simulink model "hardware_atrias_raibert"  (R2014a)
settings: Solver=FixedStepDiscrete  StartTime=0.0  StopTime=inf  FixedStep=sample_time  RelTol=1e-3
InitFcn:
  | init_hardware_atrias_raibert;
undefined symbols (not defined in the file): A_lpf_accel, A_lpf_dtau, B1_lpf_accel, B1_lpf_dtau, B2_lpf_accel, B2_lpf_dtau, boom_mount_angle, boom_mount_to_center_diagonal, boom_mount_to_com, contact_threshold, control_start_time, desired_torso_angle, DiscIntNeverNeededParam, dt_thrust, dx_avg_desired, dx_avg_samples, F_thrust, fcut_contact, g, i_limit_lateral, j_segments, k_ff, k_placement, k_sea, kd_flight, kd_lateral, kd_leg_angle, kd_sea_torque_flight, kd_sea_torque_stance, kd_torso, kd_virtual, ki_lateral, kp_flight_max, kp_flight_min, kp_lateral, kp_leg_angle, kp_sea_torque_flight, kp_sea_torque_stance, kp_torso, kp_virtual, l0_virtual, l_boom, l_max, l_min, l_retract, l_seg, lambda1, lambda2, lateral_offset, lateral_torque_ramp_time, LEG_MTR_MAX_TORQUE, loaded_threshold, m_leg_motor, m_total, max_leg_angle, max_sagittal_loaded_torque, max_sagittal_unloaded_torque, max_torque_lateral, min_leg_angle, sagittal_torque_ramp_time ... (+7)
libraries: simulink x13
settings Model: xpc_rtwmakecfg_data=_xpcethercatlib_  BufferReuse=off  Creator=wmartin  LastModifiedBy=wmartin
settings SolverCC: EnableConcurrentExecution=on
settings DataIOCC: MaxDataPoints=1000000000  SaveFormat=StructureWithTime
settings OptimizationCC: BlockReduction=off  OptimizeBlockIOStorage=off  BufferReuse=off  GlobalBufferReuse=off  ExpressionFolding=off  ExpressionDepthLimit=2147483647  LocalBlockOutputs=off
settings DebuggingCC: UnderspecifiedInitializationDetection=Classic  StateNameClashWarn=warning
settings HardwareCC: ProdIntDivRoundTo=Zero  ProdEndianess=LittleEndian  ProdHWDeviceType=Generic->32-bit x86 compatible
settings RTWCC: SystemTargetFile=slrt.tlc  TemplateMakefile=slrt_default_tmf  Description=Simulink Real-Time  RTWVerbose=off  ProcessScript=slrt_make_rtw_hook  RTWCompilerOptimization=On
settings SimulinkRealTimeCC: GeneratePreprocessorConditionals=Disable all  EnableShiftOperators=on  RL32LogBufSizeModifier=100000000

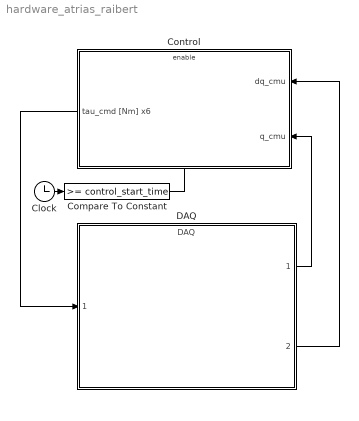
== system hardware_atrias_raibert ==
  Clock : Clock
  Compare To Constant : simulink/Logic and Bit Operations/Compare To Constant  relop=>=  const=control_start_time  OutDataTypeStr=boolean
  Control : Subsystem
  DAQ : ModelReference  ModelNameDialog=DAQ  SimulationMode=Normal  ModelReferenceVersion=1.1389  CopyOfModelName=DAQ  DefaultDataLogging=on
  wires:
  DAQ/1 -> Control/2(q_cmu)
  DAQ/2 -> Control/1(dq_cmu)
  Clock/1 -> Compare To Constant/1
  Compare To Constant/1 -> Control/Enable
  Control/1(tau_cmd [Nm] x6) -> DAQ/1

== system hardware_atrias_raibert/Control ==
  dq_cmu : Inport
  q_cmu : Inport  Port=2
  Enable : EnablePort  StatesWhenEnabling=reset
  Actuator Control : Subsystem
  Behavior Control : Subsystem
  tau_cmd [Nm] x6 : Outport  InitialOutput=[0 0 0 0 0 0]
  wires:
  Behavior Control/1(motor_torque_cmd) -> Actuator Control/1(tau_desired [Nm] x6)
  dq_cmu/1 -> Actuator Control/3(dq_cmu), Behavior Control/1(dq_cmu)
  Actuator Control/1(tau_cmd [Nm] x6) -> tau_cmd [Nm] x6/1
  q_cmu/1 -> Actuator Control/2(q_cmu), Behavior Control/2(q_cmu)

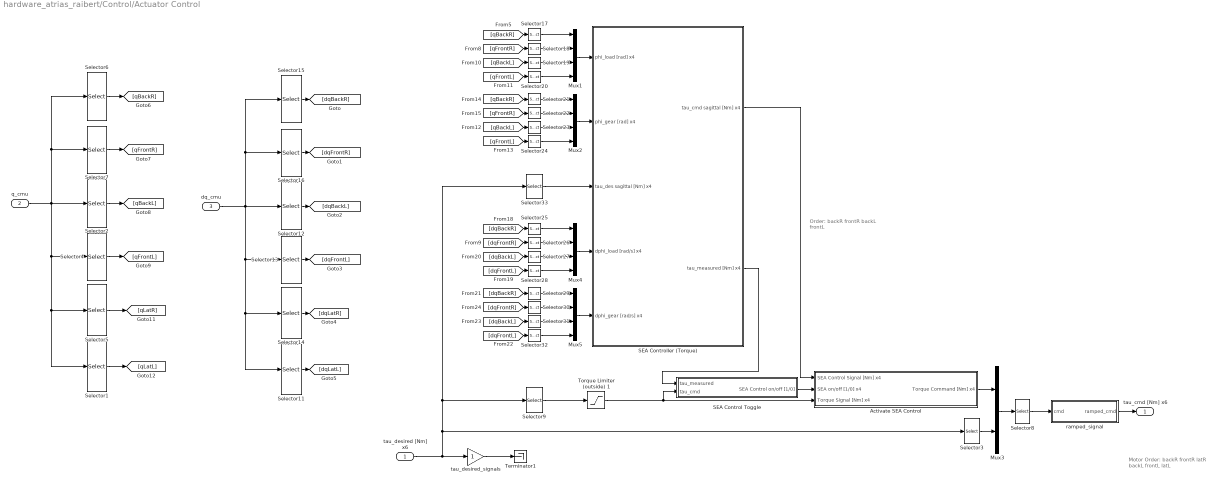
== system hardware_atrias_raibert/Control/Actuator Control ==
  note: Order:
      | backR
      | frontR
      | backL
      | frontL
  note: Motor Order:
      |
      | backR
      | frontR
      | latR
      | backL
      | frontL
      | latL
  tau_desired [Nm] x6 : Inport
  q_cmu : Inport  Port=2
  dq_cmu : Inport  Port=3
  Activate SEA Control : Subsystem
  Mux{1..2,4..5} (4 alike) : Mux
  Mux3 : Mux  Inputs=2
  SEA Control Toggle : Subsystem
  SEA Controller (Torque) : Subsystem
  Selector1 : Selector  InputPortWidth=13  Indices=[10]
  Selector11 : Selector  InputPortWidth=13  Indices=[10]
  Selector12 : Selector  InputPortWidth=13  Indices=[5 6]
  Selector13 : Selector  InputPortWidth=13  Indices=[7 8]
  Selector14 : Selector  InputPortWidth=13  Indices=[9]
  Selector15 : Selector  InputPortWidth=13  Indices=[1 2]
  Selector16 : Selector  InputPortWidth=13  Indices=[3 4]
  Selector{17..20,25..28} (8 alike) : Selector  InputPortWidth=2  Indices=[1]
  Selector2 : Selector  InputPortWidth=13  Indices=[5 6]
  Selector{21..24,29..32} (8 alike) : Selector  InputPortWidth=2  Indices=[2]
  Selector3 : Selector  InputPortWidth=6  Indices=[3 6]
  Selector33 : Selector  InputPortWidth=6  Indices=[1 2 4 5]
  Selector4 : Selector  InputPortWidth=13  Indices=[7 8]
  Selector5 : Selector  InputPortWidth=13  Indices=[9]
  Selector6 : Selector  InputPortWidth=13  Indices=[1 2]
  Selector7 : Selector  InputPortWidth=13  Indices=[3 4]
  Selector8 : Selector  InputPortWidth=6  Indices=[1 2 5 3 4 6]
  Selector9 : Selector  InputPortWidth=6  Indices=[1 2 4 5]
  Terminator1 : Terminator
  Torque Limiter (outside) 1 : Saturate  UpperLimit=max_sagittal_unloaded_torque  LowerLimit=-max_sagittal_unloaded_torque
      settings: AttributesFormatString=Hi: %<UpperLimit>\nLo: %<LowerLimit>
  ramped_signal : Subsystem
  tau_desired_signals : Gain  Description=xPCTag(1)=tau_cmd_signal;
  tau_cmd [Nm] x6 : Outport  InitialOutput=[0 0 0 0 0 0]
  wires:
  Selector9/1 -> Torque Limiter (outside) 1/1
  SEA Controller (Torque)/2(tau_measured [Nm] x4) -> SEA Control Toggle/1(tau_measured)
  SEA Control Toggle/1(SEA Control on/off [1/0]) -> Activate SEA Control/2("SEA on/off [1/0] x4 ")
  SEA Controller (Torque)/1(tau_cmd sagittal [Nm] x4) -> Activate SEA Control/1(SEA Control Signal [Nm] x4)
  Torque Limiter (outside) 1/1 -> SEA Control Toggle/2(tau_cmd), Activate SEA Control/3(Torque Signal [Nm] x4)
  Activate SEA Control/1(Torque Command [Nm] x4) -> Mux3/1
  tau_desired [Nm] x6/1 -> tau_desired_signals/1, Selector3/1, Selector9/1, Selector33/1
  ramped_signal/1(ramped_cmd) -> tau_cmd [Nm] x6/1
  tau_desired_signals/1 -> Terminator1/1
  Selector5/1 -> [qLatR]
  Selector1/1 -> [qLatL]
  Selector6/1 -> [qBackR]
  Selector7/1 -> [qFrontR]
  Selector2/1 -> [qBackL]
  Selector4/1 -> [qFrontL]
  q_cmu/1 -> Selector1/1, Selector5/1, Selector4/1, Selector6/1, Selector7/1, Selector2/1
  Selector8/1 -> ramped_signal/1(cmd)
  dq_cmu/1 -> Selector12/1, Selector16/1, Selector15/1, Selector13/1, Selector14/1, Selector11/1
  Selector14/1 -> [dqLatR]
  Selector11/1 -> [dqLatL]
  Selector15/1 -> [dqBackR]
  Selector16/1 -> [dqFrontR]
  Selector12/1 -> [dqBackL]
  Selector13/1 -> [dqFrontL]
  Mux1/1 -> SEA Controller (Torque)/1(phi_load [rad] x4)
  [qBackR] -> Selector17/1
  Selector17/1 -> Mux1/1
  Selector19/1 -> Mux1/3
  Selector18/1 -> Mux1/2
  Selector20/1 -> Mux1/4
  [qFrontR] -> Selector18/1
  [qBackL] -> Selector19/1
  [qFrontL] -> Selector20/1
  Mux2/1 -> SEA Controller (Torque)/2(phi_gear [rad] x4)
  [qBackR] -> Selector21/1
  Selector21/1 -> Mux2/1
  Selector23/1 -> Mux2/3
  Selector22/1 -> Mux2/2
  Selector24/1 -> Mux2/4
  [qFrontR] -> Selector22/1
  [qBackL] -> Selector23/1
  [qFrontL] -> Selector24/1
  Mux4/1 -> SEA Controller (Torque)/4(dphi_load [rad/s] x4)
  [dqBackR] -> Selector25/1
  Selector25/1 -> Mux4/1
  Selector27/1 -> Mux4/3
  Selector26/1 -> Mux4/2
  Selector28/1 -> Mux4/4
  [dqFrontR] -> Selector26/1
  [dqBackL] -> Selector27/1
  [dqFrontL] -> Selector28/1
  Mux5/1 -> SEA Controller (Torque)/5(dphi_gear [rad/s] x4)
  [dqBackR] -> Selector29/1
  Selector29/1 -> Mux5/1
  Selector31/1 -> Mux5/3
  Selector30/1 -> Mux5/2
  Selector32/1 -> Mux5/4
  [dqFrontR] -> Selector30/1
  [dqBackL] -> Selector31/1
  [dqFrontL] -> Selector32/1
  Selector33/1 -> SEA Controller (Torque)/3(tau_des sagittal [Nm] x4)
  Selector3/1 -> Mux3/2
  Mux3/1 -> Selector8/1

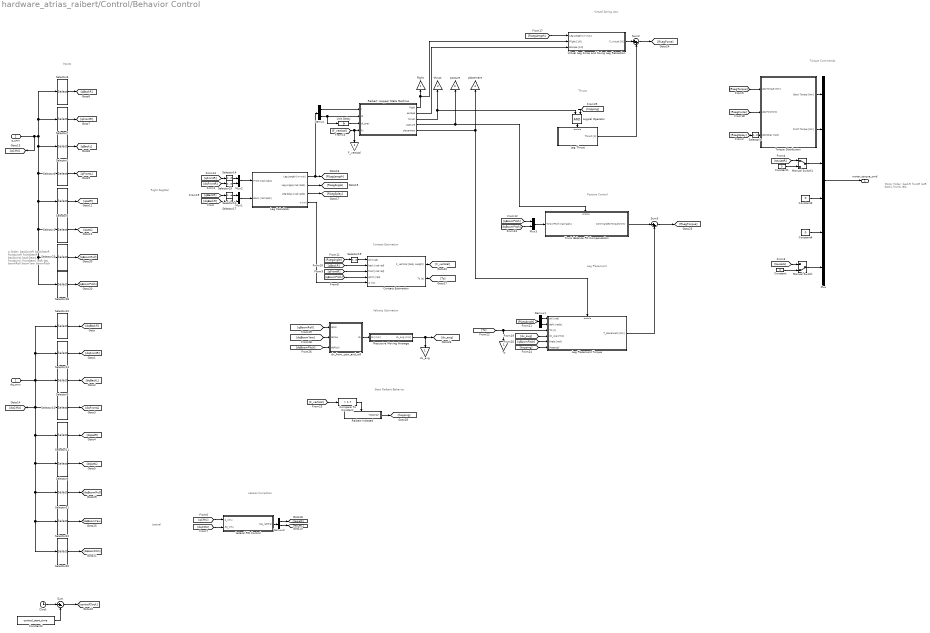
== system hardware_atrias_raibert/Control/Behavior Control ==
  note: Inputs
  note: Motor Order:
      |
      | backR
      | frontR
      | latR
      | backL
      | frontL
      | latL
  note: q Order:
      |
      | backJointR
      | backGearR
      | frontJointR
      | frontGearR
      |
      | backJointL
      | backGearL
      | frontJointL
      | frontGearL
      |
      | latR
      | latL
      |
      | boomRoll
      | boomYaw
      | boomPitch
  note: Virtual Spring Law
  note: Torque Commands
  note: Lateral
      | Correction
  note: Right Sagittal
  note: Lateral
  note: Contact Estimation
  note: Posture Control
  note: Thrust
  note: Velocity Estimation
  note: Leg Placement
  note: Start Raibert Behavior
  dq_cmu : Inport
  q_cmu : Inport  Port=2
  Clock : Clock
  Compare To Constant : simulink/Logic and Bit Operations/Compare To Constant  relop=>  const=1.7  OutDataTypeStr=boolean
  Constant{,1,3..4} (4 alike) : Constant  Value=0
  Constant2 : Constant  Value=control_start_time
  Contact Estimation : Subsystem
  Demux : Demux  Outputs=2
  Demux1 : Demux  Outputs=2
  Demux2 : Demux  Outputs=2
  F_vertical : Gain
  Lateral PID Control : Subsystem
  Leg Calculator : Subsystem
  Leg Placement Torque : Subsystem
  Leg Thrust : Subsystem
  Logical Operator : Logic  IconShape=distinctive  AllPortsSameDT=off  OutDataTypeStr=boolean
  Manual Switch : ManualSwitch  CurrentSetting=0
  Manual Switch1 : ManualSwitch
  Mux : Mux  Inputs=6
  Mux1 : Mux  Inputs=2
  Mux2 : Mux  Inputs=2
  Mux3 : Mux  Inputs=2
  Raibert  Hopper State Machine : State Transition Table  TreatAsAtomicUnit=on
  Raibert Initiated : Subsystem
  Recursive Moving Average : Subsystem
  Selector1 : Selector  InputPortWidth=13  Indices=[10]
  Selector10 : Selector  InputPortWidth=13  Indices=[7 8]
  Selector11 : Selector  InputPortWidth=13  Indices=[9]
  Selector12 : Selector  InputPortWidth=13  Indices=[1 2]
  Selector13 : Selector  InputPortWidth=13  Indices=[3 4]
  Selector{3,14..17,19} (6 alike) : Selector  InputPortWidth=2  Indices=[1]
  Selector18 : Selector  InputPortWidth=13  Indices=[13]
  Selector2 : Selector  InputPortWidth=13  Indices=[5 6]
  Selector20 : Selector  InputPortWidth=13  Indices=[13]
  Selector21 : Selector  InputPortWidth=13  Indices=[11]
  Selector22 : Selector  InputPortWidth=13  Indices=[12]
  Selector23 : Selector  InputPortWidth=13  Indices=[11]
  Selector4 : Selector  InputPortWidth=13  Indices=[7 8]
  Selector5 : Selector  InputPortWidth=13  Indices=[9]
  Selector6 : Selector  InputPortWidth=13  Indices=[1 2]
  Selector7 : Selector  InputPortWidth=13  Indices=[3 4]
  Selector8 : Selector  InputPortWidth=13  Indices=[10]
  Selector9 : Selector  InputPortWidth=13  Indices=[5 6]
  Sum : Sum  Inputs=|+-
  Sum2 : Sum  Inputs=|++
  Sum3 : Sum  Inputs=|++
  Torque Distribution : Subsystem
  Trunk Balance PD Compensation : Subsystem
  Ts : Gain
  Unit Delay : UnitDelay  SampleTime=-1
  Virtual Leg Force and Swing Leg Retraction : Subsystem
  dx_avg : Gain
  dx_from_yaw_and_roll : MATLAB Function  TreatAsAtomicUnit=on
  flight : Gain
  placement : Gain  Gain=4
  posture : Gain  Gain=3
  thrust : Gain  Gain=2
  motor_torque_cmd : Outport  OutputWhenDisabled=reset  InitialOutput=[0 0 0 0 0 0]
  wires:
  Constant4/1 -> Mux/5
  Constant3/1 -> Mux/4
  Lateral PID Control/1(tau_lateral) -> Demux2/1
  [dqCMU] -> Lateral PID Control/2(dq_cmu)
  [qCMU] -> Lateral PID Control/1(q_cmu)
  Sum/1 -> [controlClock]
  Selector4/1 -> [qFrontL]
  Selector2/1 -> [qBackL]
  Selector7/1 -> [qFrontR]
  Selector6/1 -> [qBackR]
  Selector1/1 -> [qLatL]
  Selector5/1 -> [qLatR]
  Constant2/1 -> Sum/2
  Clock/1 -> Sum/1
  Constant1/1 -> Manual Switch1/2
  Constant/1 -> Manual Switch/2
  Manual Switch/1 -> Mux/6
  Manual Switch1/1 -> Mux/3
  Mux/1 -> motor_torque_cmd/1
  Selector8/1 -> [dqLatL]
  Selector11/1 -> [dqLatR]
  Selector12/1 -> [dqBackR]
  Selector13/1 -> [dqFrontR]
  Selector9/1 -> [dqBackL]
  Selector10/1 -> [dqFrontL]
  [qBackR] -> Selector16/1
  [dqBackR] -> Selector17/1
  [qFrontR] -> Selector14/1
  [dqFrontR] -> Selector15/1
  Mux2/1 -> Leg Calculator/1(Front [rad rad/s])
  Mux1/1 -> Leg Calculator/2(Back [rad rad/s])
  Demux/1 -> Raibert  Hopper State Machine/1(l)
  Leg Calculator/1("Leg Length [m m/s] ") -> Demux/1, [RLegLength]
  Leg Calculator/2(Leg Angle [rad rad/s]) -> [RLegAngle]
  Leg Calculator/3(Leg Splay [rad rad/s]) -> [RLegSplay]
  Torque Distribution/1(Back Torque [Nm]) -> Mux/1
  Torque Distribution/2(Front Torque [Nm]) -> Mux/2
  [RLegSplay] -> Selector3/1
  Demux2/1 -> [tauLatR]
  Demux2/2 -> [tauLatL]
  [tauLatR] -> Manual Switch1/1
  [tauLatL] -> Manual Switch/1
  Selector3/1 -> Torque Distribution/3(Leg Splay [rad])
  Selector14/1 -> Mux2/1
  Selector15/1 -> Mux2/2
  Selector17/1 -> Mux1/2
  Selector16/1 -> Mux1/1
  Leg Calculator/4(w [m]) -> Contact Estimation/5(w [m])
  q_cmu/1 -> Selector6/1, Selector7/1, Selector2/1, Selector4/1, Selector5/1, Selector18/1, Selector23/1, Selector1/1, [qCMU]
  Selector18/1 -> [qBoomPitch]
  [qFrontR] -> Contact Estimation/3(front [rad rad])
  [qBackR] -> Contact Estimation/2(back [rad rad])
  [qBoomPitch] -> Contact Estimation/4(pitch [rad])
  [RLegAngle] -> Selector19/1
  Selector19/1 -> Contact Estimation/1(phi [rad])
  Contact Estimation/1(F_vertical [body weight]) -> [F_vertical]
  Raibert  Hopper State Machine/4(posture) -> Trunk Balance PD Compensation/Enable, posture/1
  Selector20/1 -> [dqBoomPitch]
  Mux3/1 -> Trunk Balance PD Compensation/1(Torso Pitch [rad rad/s])
  [qBoomPitch] -> Mux3/1
  [dqBoomPitch] -> Mux3/2
  Trunk Balance PD Compensation/1(Commanded Torque [Nm]) -> Sum3/1
  Unit Delay/1 -> Raibert  Hopper State Machine/3(dl_prev)
  [F_vertical] -> F_vertical/1, Raibert  Hopper State Machine/4(Fy)
  Demux/2 -> Unit Delay/1, Raibert  Hopper State Machine/2(dl)
  Raibert  Hopper State Machine/3(thrust) -> Logical Operator/1, thrust/1
  Leg Thrust/1(Thrust [N]) -> Sum2/2
  Sum2/1 -> [RLegForce]
  [RLegForce] -> Torque Distribution/2(Leg Force [N])
  [RLegTorque] -> Torque Distribution/1(Leg Torque [Nm])
  Raibert  Hopper State Machine/1(flight) -> flight/1, Virtual Leg Force and Swing Leg Retraction/2(Flight [1/0])
  Virtual Leg Force and Swing Leg Retraction/1(F_virtual [N]) -> Sum2/1
  [RLegLength] -> Virtual Leg Force and Swing Leg Retraction/1(Leg Length [m m/s])
  Raibert  Hopper State Machine/2(escape) -> Virtual Leg Force and Swing Leg Retraction/3(Escape [1/0])
  Selector22/1 -> [dqBoomYaw]
  Recursive Moving Average/1(dx_avg [m/s]) -> dx_avg/1, [dx_avg]
  Leg Placement Torque/1(T_placement [Nm]) -> Sum3/2
  Sum3/1 -> [RLegTorque]
  [dx_avg] -> Leg Placement Torque/4(dx_avg [m/s])
  [qBoomPitch] -> Leg Placement Torque/5(theta [rad])
  Demux1/1 -> Leg Placement Torque/1(phi [rad])
  Demux1/2 -> Leg Placement Torque/2(dphi [rad/s])
  [RLegAngle] -> Demux1/1
  [Ts] -> Leg Placement Torque/3(Ts [s]), Ts/1
  Contact Estimation/2(Ts [s]) -> [Ts]
  Raibert  Hopper State Machine/5(placement) -> Leg Placement Torque/Enable, placement/1
  [F_vertical] -> Compare To Constant/1
  Compare To Constant/1 -> Raibert Initiated/Enable
  Raibert Initiated/1(Hopping?) -> [hopping]
  [hopping] -> Leg Placement Torque/6(Hopping?)
  Logical Operator/1 -> Leg Thrust/Enable
  [hopping] -> Logical Operator/2
  dx_from_yaw_and_roll/1(dx) -> Recursive Moving Average/1(dx [m/s])
  [dqBoomYaw] -> dx_from_yaw_and_roll/2(dqYaw)
  dq_cmu/1 -> Selector20/1, Selector22/1, Selector21/1, Selector8/1, Selector11/1, Selector10/1, [dqCMU], Selector12/1, Selector13/1, Selector9/1
  Selector21/1 -> [dqBoomRoll]
  Selector23/1 -> [qBoomRoll]
  [qBoomRoll] -> dx_from_yaw_and_roll/1(qRoll)
  [dqBoomPitch] -> dx_from_yaw_and_roll/3(dqPitch)

== system hardware_atrias_raibert/Control/Actuator Control/Activate SEA Control ==
  SEA Control Signal [Nm] x4 : Inport
  "SEA on/off [1/0] x4 " : Inport  Port=2
  Torque Signal [Nm] x4 : Inport  Port=3
  Demux : Demux
  Demux2 : Demux
  Demux3 : Demux
  Mux6 : Mux
  Switch{,1..3} (4 alike) : Switch  Criteria=u2 ~= 0
  Torque Command [Nm] x4 : Outport
  wires:
  Torque Signal [Nm] x4/1 -> Demux2/1
  "SEA on/off [1/0] x4 "/1 -> Demux3/1
  SEA Control Signal [Nm] x4/1 -> Demux/1
  Demux2/3 -> Switch2/3
  Demux/2 -> Switch1/1
  Demux3/4 -> Switch3/2
  Demux2/4 -> Switch3/3
  Demux/4 -> Switch3/1
  Switch2/1 -> Mux6/3
  Demux/3 -> Switch2/1
  Demux3/2 -> Switch1/2
  Demux3/3 -> Switch2/2
  Mux6/1 -> Torque Command [Nm] x4/1
  Demux3/1 -> Switch/2
  Switch3/1 -> Mux6/4
  Switch1/1 -> Mux6/2
  Switch/1 -> Mux6/1
  Demux/1 -> Switch/1
  Demux2/1 -> Switch/3
  Demux2/2 -> Switch1/3

== system hardware_atrias_raibert/Control/Actuator Control/SEA Control Toggle ==
  tau_measured : Inport
  tau_cmd : Inport  Port=2
  Abs : Abs
  Abs1 : Abs
  But Commanding a Small Torque? : simulink/Logic and Bit Operations/Compare To Constant  relop=<  const=sea_control_torque_cmd_small_threshold  OutDataTypeStr=boolean
  Logical Operator1 : Logic  AllPortsSameDT=off  OutDataTypeStr=boolean
  Logical Operator2 : Logic  Operator=NOT  AllPortsSameDT=off  OutDataTypeStr=boolean
  Measuring a Large Torque? (High Gains) : simulink/Logic and Bit Operations/Compare To Constant  relop=>=  const=stance_flight_torque_threshold  OutDataTypeStr=boolean
  SEA Control on/off [1/0] : Outport
  wires:
  Abs1/1 -> Measuring a Large Torque? (High Gains)/1
  Measuring a Large Torque? (High Gains)/1 -> Logical Operator1/1
  tau_measured/1 -> Abs1/1
  Abs/1 -> But Commanding a Small Torque?/1
  tau_cmd/1 -> Abs/1
  Logical Operator1/1 -> Logical Operator2/1
  But Commanding a Small Torque?/1 -> Logical Operator1/2
  Logical Operator2/1 -> SEA Control on/off [1/0]/1

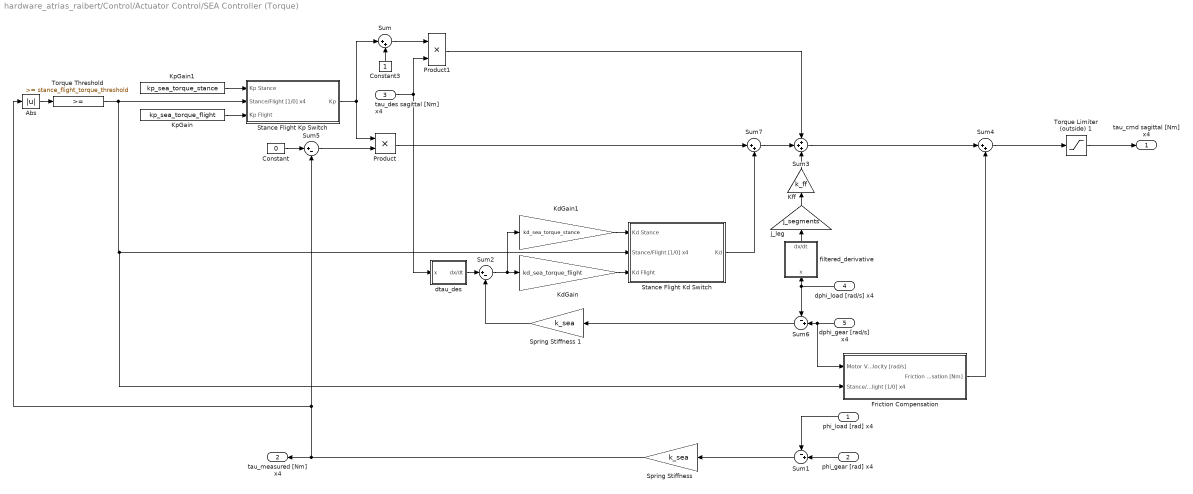
== system hardware_atrias_raibert/Control/Actuator Control/SEA Controller (Torque) ==
  phi_load [rad] x4 : Inport
  phi_gear [rad] x4 : Inport  Port=2
  tau_des sagittal [Nm] x4 : Inport  Port=3
  dphi_load [rad/s] x4 : Inport  Port=4
  dphi_gear [rad/s] x4 : Inport  Port=5
  Abs : Abs
  Constant : Constant  Value=0
  Constant3 : Constant
  Friction Compensation : Subsystem
  KdGain : Gain  Description=xPCTag(1)=kd_sea_torque;  Gain=kd_sea_torque_flight
  KdGain1 : Gain  Description=xPCTag(1)=kd_sea_torque;  Gain=kd_sea_torque_stance
  Kff : Gain  Gain=k_ff
  KpGain : Constant  Value=kp_sea_torque_flight  SampleTime=sample_time
  KpGain1 : Constant  Value=kp_sea_torque_stance  SampleTime=sample_time
  Product : Product  SampleTime=sample_time  RndMeth=Zero
  Product1 : Product  RndMeth=Zero
  Spring Stiffness : Gain  Gain=k_sea
  Spring Stiffness 1 : Gain  Gain=k_sea
  Stance Flight Kd Switch : Subsystem
  Stance Flight Kp Switch : Subsystem
  Sum : Sum  Inputs=|++  SampleTime=sample_time
  Sum1 : Sum  Inputs=-+|
  Sum2 : Sum  Inputs=|+-
  Sum3 : Sum  Inputs=+++
  Sum4 : Sum  Inputs=|++
  Sum5 : Sum  Inputs=|+-
  Sum6 : Sum  Inputs=-+|
  Sum7 : Sum  Inputs=|++
  Torque Limiter (outside) 1 : Saturate  UpperLimit=max_sagittal_loaded_torque  LowerLimit=-max_sagittal_loaded_torque
      settings: AttributesFormatString=Hi: %<UpperLimit>\nLo: %<LowerLimit>
  Torque Threshold : simulink/Logic and Bit Operations/Compare To Constant  relop=>=  const=stance_flight_torque_threshold  OutDataTypeStr=boolean
  dtau_des : Subsystem
  filtered_derivative : Subsystem
  j_leg : Gain  Description=xPCTag(1)=kd_sea_torque;  Gain=j_segments
  tau_cmd sagittal [Nm] x4 : Outport
  tau_measured [Nm] x4 : Outport  Port=2
  wires:
  Kff/1 -> Sum3/3
  Torque Limiter (outside) 1/1 -> tau_cmd sagittal [Nm] x4/1
  j_leg/1 -> Kff/1
  filtered_derivative/1(dx/dt) -> j_leg/1
  Sum/1 -> Product1/1
  Constant3/1 -> Sum/2
  Sum7/1 -> Sum3/2
  KdGain/1 -> Stance Flight Kd Switch/3(Kd Flight)
  Product/1 -> Sum7/1
  Sum5/1 -> Product/2
  Sum2/1 -> KdGain1/1, KdGain/1
  dphi_gear [rad/s] x4/1 -> Friction Compensation/1(Motor Velocity [rad/s]), Sum6/2
  dphi_load [rad/s] x4/1 -> filtered_derivative/1(x), Sum6/1
  Spring Stiffness 1/1 -> Sum2/2
  Sum6/1 -> Spring Stiffness 1/1
  dtau_des/1(dx/dt) -> Sum2/1
  Constant/1 -> Sum5/1
  phi_gear [rad] x4/1 -> Sum1/2
  phi_load [rad] x4/1 -> Sum1/1
  Product1/1 -> Sum3/1
  tau_des sagittal [Nm] x4/1 -> Product1/2, dtau_des/1(x)
  Sum1/1 -> Spring Stiffness/1
  KpGain1/1 -> Stance Flight Kp Switch/1(Kp Stance)
  Torque Threshold/1 -> Friction Compensation/2(Stance/Flight [1/0] x4), Stance Flight Kd Switch/2(Stance/Flight [1/0] x4), Stance Flight Kp Switch/2(Stance/Flight [1/0] x4)
  KpGain/1 -> Stance Flight Kp Switch/3(Kp Flight)
  KdGain1/1 -> Stance Flight Kd Switch/1(Kd Stance)
  Spring Stiffness/1 -> Sum5/2, Abs/1, tau_measured [Nm] x4/1
  Stance Flight Kp Switch/1(Kp) -> Sum/1, Product/1
  Abs/1 -> Torque Threshold/1
  Sum3/1 -> Sum4/1
  Friction Compensation/1(Friction Compensation [Nm]) -> Sum4/2
  Sum4/1 -> Torque Limiter (outside) 1/1
  Stance Flight Kd Switch/1(Kd) -> Sum7/2

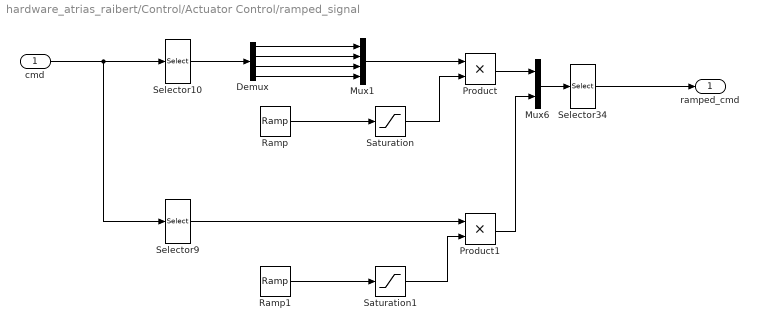
== system hardware_atrias_raibert/Control/Actuator Control/ramped_signal ==
  cmd : Inport
  Demux : Demux
  Mux1 : Mux
  Mux6 : Mux  Inputs=2
  Product : Product  RndMeth=Zero
  Product1 : Product  RndMeth=Zero
  Ramp : simulink/Sources/Ramp  slope=1/sagittal_torque_ramp_time  start=sagittal_starting_time  X0=0
      settings: AttributesFormatString=Start: %<start>\nSlope: %<slope>
  Ramp1 : simulink/Sources/Ramp  slope=1/lateral_torque_ramp_time  start=control_start_time  X0=0
      settings: AttributesFormatString=Start: %<start>\nSlope: %<slope>
  Saturation : Saturate  UpperLimit=1  LowerLimit=0
      settings: AttributesFormatString=Hi: %<UpperLimit>\nLo: %<LowerLimit>
  Saturation1 : Saturate  UpperLimit=1  LowerLimit=0
      settings: AttributesFormatString=Hi: %<UpperLimit>\nLo: %<LowerLimit>
  Selector10 : Selector  InputPortWidth=6  Indices=[1 2 4 5]
  Selector34 : Selector  InputPortWidth=6  Indices=[1 2 5 3 4 6]
  Selector9 : Selector  InputPortWidth=6  Indices=[3 6]
  ramped_cmd : Outport
  wires:
  Demux/3 -> Mux1/3
  Demux/4 -> Mux1/4
  Mux1/1 -> Product/1
  Demux/2 -> Mux1/2
  Demux/1 -> Mux1/1
  Mux6/1 -> Selector34/1
  Selector10/1 -> Demux/1
  Selector34/1 -> ramped_cmd/1
  Product1/1 -> Mux6/2
  cmd/1 -> Selector9/1, Selector10/1
  Product/1 -> Mux6/1
  Ramp/1 -> Saturation/1
  Saturation/1 -> Product/2
  Ramp1/1 -> Saturation1/1
  Saturation1/1 -> Product1/2
  Selector9/1 -> Product1/1

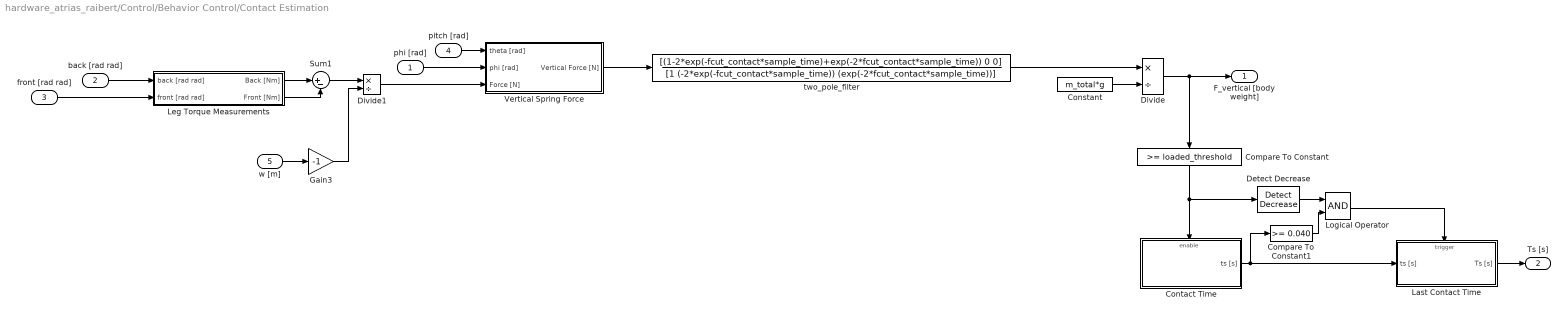
== system hardware_atrias_raibert/Control/Behavior Control/Contact Estimation ==
  phi [rad] : Inport
  back [rad rad] : Inport  Port=2
  front [rad rad] : Inport  Port=3
  pitch [rad] : Inport  Port=4
  w [m] : Inport  Port=5
  Compare To Constant : simulink/Logic and Bit Operations/Compare To Constant  relop=>=  const=loaded_threshold  OutDataTypeStr=boolean
  Compare To Constant1 : simulink/Logic and Bit Operations/Compare To Constant  relop=>=  const=0.040  OutDataTypeStr=boolean
  Constant : Constant  Value=m_total*g
  Contact Time : Subsystem
  Detect Decrease : simulink/Logic and Bit Operations/Detect Decrease  vinit=0.0  InputProcessing=Inherited  OutDataTypeStr=boolean
  Divide : Product  Inputs=*/
  Divide1 : Product  Inputs=*/
  Gain3 : Gain  Gain=-1
  Last Contact Time : Subsystem
  Leg Torque Measurements : Subsystem
  Logical Operator : Logic  AllPortsSameDT=off  OutDataTypeStr=boolean
  Sum1 : Sum  Inputs=|+-
  Vertical Spring Force : Subsystem
  two_pole_filter : DiscreteTransferFcn  Numerator=[(1-2*exp(-fcut_contact*sample_time)+exp(-2*fcut_contact*sample_time)) 0 0]  Denominator=[1 (-2*exp(-fcut_contact*sample_time)) (exp(-2*fcut_contact*sample_time))]  SampleTime=sample_time
  F_vertical [body weight] : Outport
  Ts [s] : Outport  Port=2
  wires:
  Vertical Spring Force/1(Vertical Force [N]) -> two_pole_filter/1
  Constant/1 -> Divide/2
  two_pole_filter/1 -> Divide/1
  back [rad rad]/1 -> Leg Torque Measurements/1(back [rad rad])
  Leg Torque Measurements/1(Back [Nm]) -> Sum1/1
  Leg Torque Measurements/2(Front [Nm]) -> Sum1/2
  Sum1/1 -> Divide1/1
  Divide1/1 -> Vertical Spring Force/3(Force [N])
  pitch [rad]/1 -> Vertical Spring Force/1(theta [rad])
  w [m]/1 -> Gain3/1
  Gain3/1 -> Divide1/2
  front [rad rad]/1 -> Leg Torque Measurements/2(front [rad rad])
  phi [rad]/1 -> Vertical Spring Force/2(phi [rad])
  Last Contact Time/1(Ts [s]) -> Ts [s]/1
  Contact Time/1(ts [s]) -> Last Contact Time/1(ts [s]), Compare To Constant1/1
  Compare To Constant/1 -> Detect Decrease/1, Contact Time/Enable
  Divide/1 -> F_vertical [body weight]/1, Compare To Constant/1
  Logical Operator/1 -> Last Contact Time/Trigger
  Detect Decrease/1 -> Logical Operator/1
  Compare To Constant1/1 -> Logical Operator/2

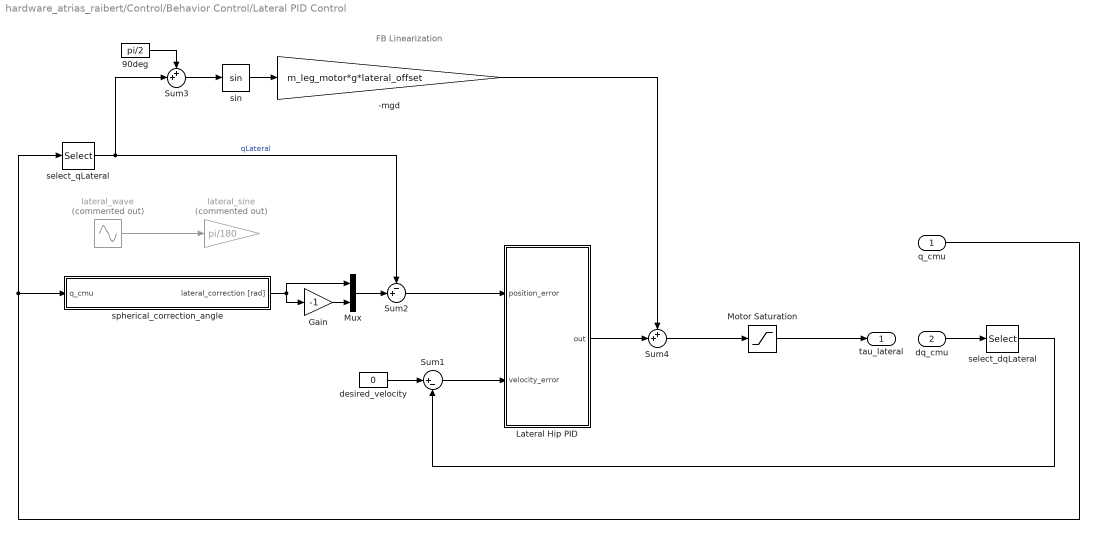
== system hardware_atrias_raibert/Control/Behavior Control/Lateral PID Control ==
  note: FB Linearization
  q_cmu : Inport
  dq_cmu : Inport  Port=2
  -mgd : Gain  Gain=m_leg_motor*g*lateral_offset
  90deg : Constant  Value=pi/2
  Gain : Gain  Gain=-1
  Lateral Hip PID : Subsystem
  Motor Saturation : Saturate  UpperLimit=max_torque_lateral  LowerLimit=-max_torque_lateral
      settings: AttributesFormatString=Top: %<UpperLimit>\nBottom: %<LowerLimit>
  Mux : Mux  Inputs=2
  Sum1 : Sum  Inputs=|+-
  Sum2 : Sum  Inputs=-+|
  Sum3 : Sum  Inputs=++|
  Sum4 : Sum  Inputs=++|
  desired_velocity : Constant  Value=0
  lateral_sine : Gain  Commented=on  Gain=pi/180
  lateral_wave : Sin  Commented=on  Amplitude=5  Frequency=2*pi*(1/2)  SampleTime=0
  select_dqLateral : Selector  InputPortWidth=13  Indices=[9 10]
  select_qLateral : Selector  InputPortWidth=13  Indices=[9 10]
  sin : Trigonometry
  spherical_correction_angle : Subsystem
  tau_lateral : Outport
  wires:
  lateral_wave/1 -> lateral_sine/1
  Lateral Hip PID/1(out) -> Sum4/2
  Sum2/1 -> Lateral Hip PID/1(position_error)
  q_cmu/1 -> spherical_correction_angle/1(q_cmu), select_qLateral/1
  select_dqLateral/1 -> Sum1/2
  dq_cmu/1 -> select_dqLateral/1
  Sum4/1 -> Motor Saturation/1
  desired_velocity/1 -> Sum1/1
  Sum1/1 -> Lateral Hip PID/2(velocity_error)
  Gain/1 -> Mux/2
  Mux/1 -> Sum2/2
  select_qLateral/1 -> Sum3/2, Sum2/1  "qLateral"
  Motor Saturation/1 -> tau_lateral/1
  spherical_correction_angle/1(lateral_correction [rad]) -> Mux/1, Gain/1
  -mgd/1 -> Sum4/1
  Sum3/1 -> sin/1
  90deg/1 -> Sum3/1
  sin/1 -> -mgd/1

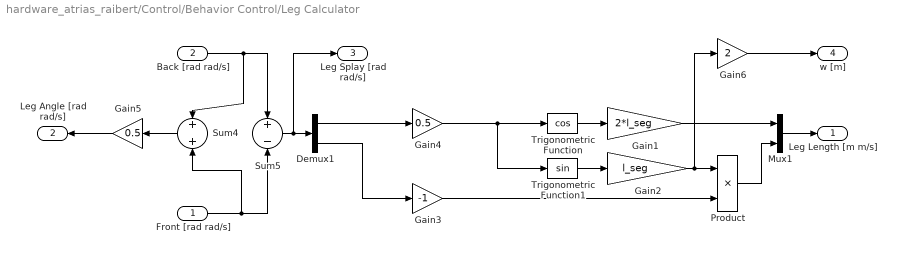
== system hardware_atrias_raibert/Control/Behavior Control/Leg Calculator ==
  Front [rad rad/s] : Inport
  Back [rad rad/s] : Inport  Port=2
  Demux1 : Demux  Outputs=2
  Gain1 : Gain  Gain=2*l_seg
  Gain2 : Gain  Gain=l_seg
  Gain3 : Gain  Gain=-1
  Gain4 : Gain  Gain=0.5
  Gain5 : Gain  Gain=0.5
  Gain6 : Gain  Gain=2
  Mux1 : Mux  Inputs=2
  Product : Product  RndMeth=Zero
  Sum4 : Sum  Inputs=+|+
  Sum5 : Sum  Inputs=+|-
  Trigonometric Function : Trigonometry  Operator=cos
  Trigonometric Function1 : Trigonometry
  "Leg Length [m m/s] " : Outport
  Leg Angle [rad rad/s] : Outport  Port=2
  Leg Splay [rad rad/s] : Outport  Port=3
  w [m] : Outport  Port=4
  wires:
  Gain6/1 -> w [m]/1
  Gain4/1 -> Trigonometric Function1/1, Trigonometric Function/1
  Trigonometric Function/1 -> Gain1/1
  Gain1/1 -> Mux1/1
  Trigonometric Function1/1 -> Gain2/1
  Product/1 -> Mux1/2
  Front [rad rad/s]/1 -> Sum5/2, Sum4/2
  Back [rad rad/s]/1 -> Sum4/1, Sum5/1
  Demux1/2 -> Gain3/1
  Gain3/1 -> Product/2
  Demux1/1 -> Gain4/1
  Gain2/1 -> Product/1, Gain6/1
  Sum5/1 -> Leg Splay [rad rad/s]/1, Demux1/1
  Mux1/1 -> "Leg Length [m m/s] "/1
  Sum4/1 -> Gain5/1
  Gain5/1 -> Leg Angle [rad rad/s]/1

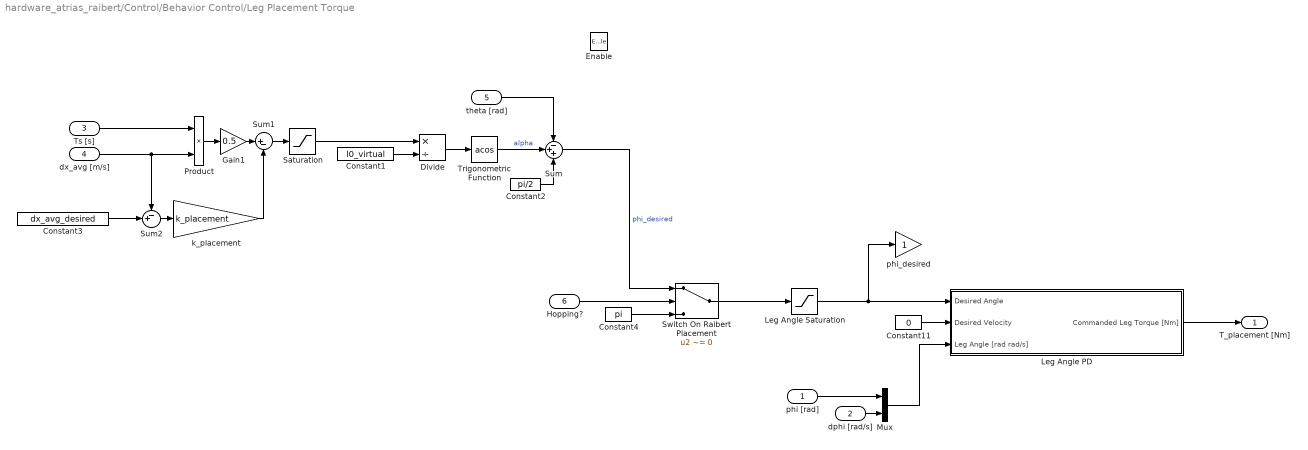
== system hardware_atrias_raibert/Control/Behavior Control/Leg Placement Torque ==
  phi [rad] : Inport
  dphi [rad/s] : Inport  Port=2
  Ts [s] : Inport  Port=3
  dx_avg [m/s] : Inport  Port=4
  theta [rad] : Inport  Port=5
  Hopping? : Inport  Port=6
  Enable : EnablePort  StatesWhenEnabling=reset
  Constant1 : Constant  Value=l0_virtual
  Constant11 : Constant  Value=0
  Constant2 : Constant  Value=pi/2
  Constant3 : Constant  Value=dx_avg_desired
  Constant4 : Constant  Value=pi
  Divide : Product  Inputs=*/
  Gain1 : Gain  Gain=0.5
  Leg Angle PD : Subsystem
  Leg Angle Saturation : Saturate  UpperLimit=max_leg_angle  LowerLimit=min_leg_angle
      settings: AttributesFormatString=Hi: %<UpperLimit>\nLo: %<LowerLimit>
  Mux : Mux  Inputs=2
  Product : Product
  Saturation : Saturate  UpperLimit=x_limit  LowerLimit=-x_limit
      settings: AttributesFormatString=Hi: %<UpperLimit>\nLo: %<LowerLimit>
  Sum : Sum  Inputs=-++
  Sum1 : Sum  Inputs=|+-
  Sum2 : Sum  Inputs=-+|
  Switch On Raibert Placement : Switch  Criteria=u2 ~= 0
  Trigonometric Function : Trigonometry  Operator=acos
  k_placement : Gain  Gain=k_placement
  phi_desired : Gain
  T_placement [Nm] : Outport  OutputWhenDisabled=reset  InitialOutput=[0]
  wires:
  Constant11/1 -> Leg Angle PD/2(Desired Velocity)
  Mux/1 -> Leg Angle PD/3(Leg Angle [rad rad/s])
  Leg Angle PD/1(Commanded Leg Torque [Nm]) -> T_placement [Nm]/1
  phi [rad]/1 -> Mux/1
  dphi [rad/s]/1 -> Mux/2
  Ts [s]/1 -> Product/1
  Product/1 -> Gain1/1
  Gain1/1 -> Sum1/1
  Saturation/1 -> Divide/1
  Constant1/1 -> Divide/2
  Divide/1 -> Trigonometric Function/1
  Trigonometric Function/1 -> Sum/2  "alpha"
  Constant2/1 -> Sum/3
  theta [rad]/1 -> Sum/1
  Sum/1 -> Switch On Raibert Placement/1  "phi_desired"
  Sum1/1 -> Saturation/1
  k_placement/1 -> Sum1/2
  Sum2/1 -> k_placement/1
  Constant3/1 -> Sum2/2
  dx_avg [m/s]/1 -> Sum2/1, Product/2
  Switch On Raibert Placement/1 -> Leg Angle Saturation/1
  Constant4/1 -> Switch On Raibert Placement/3
  Hopping?/1 -> Switch On Raibert Placement/2
  Leg Angle Saturation/1 -> phi_desired/1, Leg Angle PD/1(Desired Angle)

== system hardware_atrias_raibert/Control/Behavior Control/Leg Thrust ==
  Enable : EnablePort  StatesWhenEnabling=reset  ShowOutputPort=on
  F_thrust : Gain  Gain=F_thrust
  Thrust Timer : Subsystem
  thrust period? : simulink/Logic and Bit Operations/Compare To Constant  relop=<=  const=dt_thrust  OutDataTypeStr=uint8
  Thrust [N] : Outport  OutputWhenDisabled=reset  InitialOutput=[0]
  wires:
  F_thrust/1 -> Thrust [N]/1
  Thrust Timer/1(timer [s]) -> thrust period?/1
  Enable/1 -> Thrust Timer/Enable
  thrust period?/1 -> F_thrust/1

== system hardware_atrias_raibert/Control/Behavior Control/Raibert Initiated ==
  Enable : EnablePort  StatesWhenEnabling=reset
  Constant : Constant
  Hopping? : Outport  InitialOutput=[0]
  wires:
  Constant/1 -> Hopping?/1

== system hardware_atrias_raibert/Control/Behavior Control/Recursive Moving Average ==
  dx [m/s] : Inport
  Delay : Delay  DelayLength=dx_avg_samples  InitialCondition=0  UseCircularBuffer=on  SampleTime=sample_time
  Gain : Gain  Gain=1/dx_avg_samples
  Sum : Sum  Inputs=-++
  Unit Delay : UnitDelay  SampleTime=sample_time
  dx_avg [m/s] : Outport
  wires:
  dx [m/s]/1 -> Delay/1, Sum/2
  Sum/1 -> Gain/1, Unit Delay/1
  Delay/1 -> Sum/1
  Gain/1 -> dx_avg [m/s]/1
  Unit Delay/1 -> Sum/3

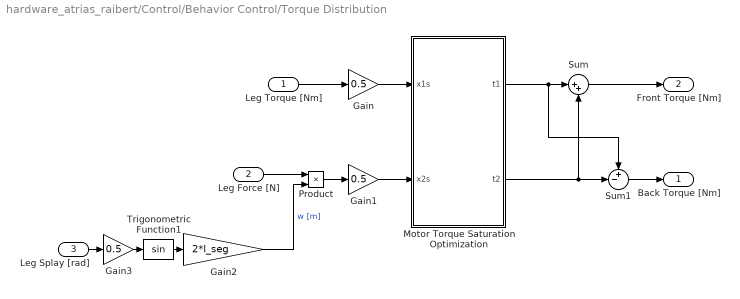
== system hardware_atrias_raibert/Control/Behavior Control/Torque Distribution ==
  Leg Torque [Nm] : Inport
  Leg Force [N] : Inport  Port=2
  Leg Splay [rad] : Inport  Port=3
  Gain : Gain  Gain=0.5
  Gain1 : Gain  Gain=0.5
  Gain2 : Gain  Gain=2*l_seg
  Gain3 : Gain  Gain=0.5
  Motor Torque Saturation Optimization : MATLAB Function  TreatAsAtomicUnit=on
  Product : Product  RndMeth=Zero
  Sum : Sum  Inputs=|++
  Sum1 : Sum  Inputs=+-|
  Trigonometric Function1 : Trigonometry
  Back Torque [Nm] : Outport
  Front Torque [Nm] : Outport  Port=2
  wires:
  Sum1/1 -> Back Torque [Nm]/1
  Leg Torque [Nm]/1 -> Gain/1
  Sum/1 -> Front Torque [Nm]/1
  Motor Torque Saturation Optimization/1(t1) -> Sum/1, Sum1/1
  Gain3/1 -> Trigonometric Function1/1
  Leg Splay [rad]/1 -> Gain3/1
  Trigonometric Function1/1 -> Gain2/1
  Gain2/1 -> Product/2  "w [m]"
  Motor Torque Saturation Optimization/2(t2) -> Sum1/2, Sum/2
  Leg Force [N]/1 -> Product/1
  Product/1 -> Gain1/1
  Gain1/1 -> Motor Torque Saturation Optimization/2(x2s)
  Gain/1 -> Motor Torque Saturation Optimization/1(x1s)

== system hardware_atrias_raibert/Control/Behavior Control/Trunk Balance PD Compensation ==
  Torso Pitch [rad rad/s] : Inport
  Enable : EnablePort  StatesWhenEnabling=reset
  Constant2 : Constant  Value=0
  Demux : Demux  Outputs=2
  Derivative Gain : Gain  Gain=kd_torso
  Gain1 : Gain  Gain=-1
  Proportional Gain : Gain  Gain=kp_torso
  Reference Lean [rad] : Constant  Value=desired_torso_angle
  Sum1 : Sum  Inputs=|+-
  Sum4 : Sum  Inputs=|+-
  Sum5 : Sum
  Commanded Torque [Nm] : Outport  OutputWhenDisabled=reset  InitialOutput=[0]
  wires:
  Gain1/1 -> Commanded Torque [Nm]/1
  Sum1/1 -> Derivative Gain/1
  Proportional Gain/1 -> Sum5/1
  Derivative Gain/1 -> Sum5/2
  Torso Pitch [rad rad/s]/1 -> Demux/1
  Sum4/1 -> Proportional Gain/1
  Demux/1 -> Sum4/2
  Reference Lean [rad]/1 -> Sum4/1
  Constant2/1 -> Sum1/1
  Demux/2 -> Sum1/2
  Sum5/1 -> Gain1/1

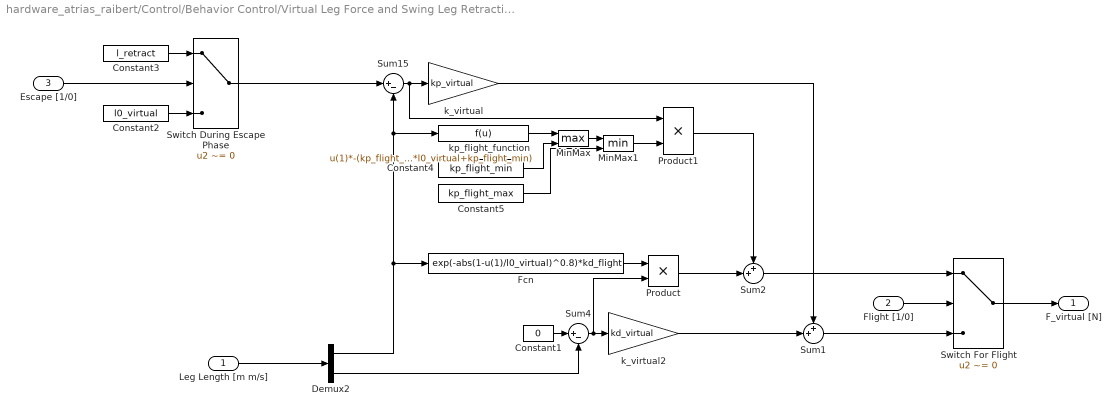
== system hardware_atrias_raibert/Control/Behavior Control/Virtual Leg Force and Swing Leg Retraction ==
  Leg Length [m m/s] : Inport
  Flight [1/0] : Inport  Port=2
  Escape [1/0] : Inport  Port=3
  Constant1 : Constant  Value=0
  Constant2 : Constant  Value=l0_virtual
  Constant3 : Constant  Value=l_retract
  Constant4 : Constant  Value=kp_flight_min
  Constant5 : Constant  Value=kp_flight_max
  Demux2 : Demux  Outputs=2
  Fcn : Fcn  Expr=exp(-abs(1-u(1)/l0_virtual)^0.8)*kd_flight
  MinMax : MinMax  Function=max  Inputs=2
  MinMax1 : MinMax  Inputs=2
  Product : Product
  Product1 : Product
  Sum1 : Sum  Inputs=++|
  Sum15 : Sum  Inputs=|+-
  Sum2 : Sum  Inputs=++|
  Sum4 : Sum  Inputs=|+-
  Switch During Escape Phase : Switch  Criteria=u2 ~= 0
  Switch For Flight : Switch  Criteria=u2 ~= 0
  k_virtual : Gain  Gain=kp_virtual
  k_virtual2 : Gain  Gain=kd_virtual
  kp_flight_function : Fcn  Expr=u(1)*-(kp_flight_max - kp_flight_min)/(l0_virtual - l_min)+((kp_flight_max - kp_flight_min)/(l0_virtual - l_min)*l0_virtual+kp_flight_min)
  F_virtual [N] : Outport
  wires:
  Sum2/1 -> Switch For Flight/1
  Switch For Flight/1 -> F_virtual [N]/1
  Product/1 -> Sum2/2
  Constant3/1 -> Switch During Escape Phase/1
  Constant2/1 -> Switch During Escape Phase/3
  Escape [1/0]/1 -> Switch During Escape Phase/2
  Flight [1/0]/1 -> Switch For Flight/2
  k_virtual2/1 -> Sum1/2
  Sum4/1 -> Product/2, k_virtual2/1
  k_virtual/1 -> Sum1/1
  Demux2/2 -> Sum4/2
  Constant1/1 -> Sum4/1
  Sum1/1 -> Switch For Flight/3
  Demux2/1 -> kp_flight_function/1, Sum15/2, Fcn/1
  Leg Length [m m/s]/1 -> Demux2/1
  Sum15/1 -> Product1/1, k_virtual/1
  Switch During Escape Phase/1 -> Sum15/1
  Fcn/1 -> Product/1
  kp_flight_function/1 -> MinMax/1
  Product1/1 -> Sum2/1
  MinMax/1 -> MinMax1/1
  Constant4/1 -> MinMax/2
  MinMax1/1 -> Product1/2
  Constant5/1 -> MinMax1/2

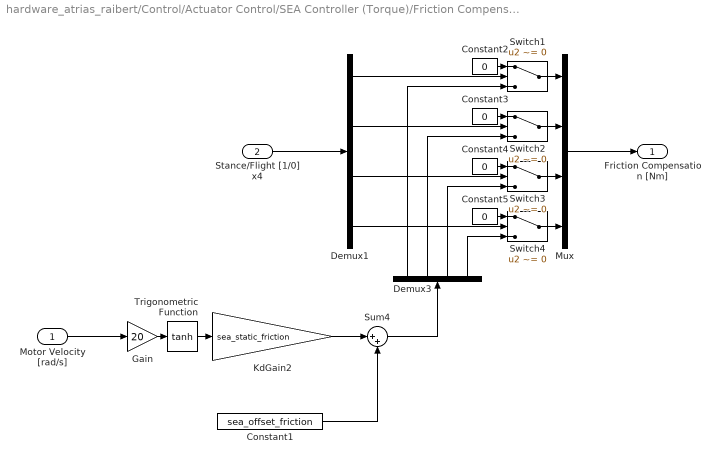
== system hardware_atrias_raibert/Control/Actuator Control/SEA Controller (Torque)/Friction Compensation ==
  Motor Velocity [rad/s] : Inport
  Stance/Flight [1/0] x4 : Inport  Port=2
  Constant1 : Constant  Value=sea_offset_friction
  Constant{2..5} (4 alike) : Constant  Value=0
  Demux1 : Demux
  Demux3 : Demux
  Gain : Gain  Gain=20
  KdGain2 : Gain  Description=xPCTag(1)=kd_sea_torque;  Gain=sea_static_friction
  Mux : Mux
  Sum4 : Sum  Inputs=|++
  Switch{1..4} (4 alike) : Switch  Criteria=u2 ~= 0
  Trigonometric Function : Trigonometry  Operator=tanh
  Friction Compensation [Nm] : Outport
  wires:
  Constant1/1 -> Sum4/2
  KdGain2/1 -> Sum4/1
  Trigonometric Function/1 -> KdGain2/1
  Gain/1 -> Trigonometric Function/1
  Motor Velocity [rad/s]/1 -> Gain/1
  Demux1/4 -> Switch4/2
  Demux1/3 -> Switch3/2
  Demux1/2 -> Switch2/2
  Switch2/1 -> Mux/2
  Switch3/1 -> Mux/3
  Switch4/1 -> Mux/4
  Switch1/1 -> Mux/1
  Demux1/1 -> Switch1/2
  Demux3/4 -> Switch4/3
  Demux3/3 -> Switch3/3
  Demux3/2 -> Switch2/3
  Demux3/1 -> Switch1/3
  Stance/Flight [1/0] x4/1 -> Demux1/1
  Constant2/1 -> Switch1/1
  Constant3/1 -> Switch2/1
  Constant4/1 -> Switch3/1
  Constant5/1 -> Switch4/1
  Sum4/1 -> Demux3/1
  Mux/1 -> Friction Compensation [Nm]/1

== system hardware_atrias_raibert/Control/Actuator Control/SEA Controller (Torque)/Stance Flight Kd Switch ==
  Kd Stance : Inport
  Stance/Flight [1/0] x4 : Inport  Port=2
  Kd Flight : Inport  Port=3
  Demux : Demux
  Demux1 : Demux
  Demux2 : Demux
  Mux : Mux
  Switch{,1..3} (4 alike) : Switch  Criteria=u2 ~= 0
  Kd : Outport
  wires:
  Demux/4 -> Switch3/2
  Demux/3 -> Switch2/2
  Demux/2 -> Switch1/2
  Switch1/1 -> Mux/2
  Switch2/1 -> Mux/3
  Switch3/1 -> Mux/4
  Stance/Flight [1/0] x4/1 -> Demux/1
  Mux/1 -> Kd/1
  Switch/1 -> Mux/1
  Demux/1 -> Switch/2
  Kd Stance/1 -> Demux1/1
  Demux1/1 -> Switch/1
  Demux1/2 -> Switch1/1
  Demux1/3 -> Switch2/1
  Demux1/4 -> Switch3/1
  Kd Flight/1 -> Demux2/1
  Demux2/4 -> Switch3/3
  Demux2/3 -> Switch2/3
  Demux2/2 -> Switch1/3
  Demux2/1 -> Switch/3

== system hardware_atrias_raibert/Control/Actuator Control/SEA Controller (Torque)/Stance Flight Kp Switch ==
  Kp Stance : Inport
  Stance/Flight [1/0] x4 : Inport  Port=2
  Kp Flight : Inport  Port=3
  Demux : Demux
  Mux : Mux
  Switch{,1..3} (4 alike) : Switch  Criteria=u2 ~= 0
  Kp : Outport
  wires:
  Kp Flight/1 -> Switch/3, Switch3/3, Switch2/3, Switch1/3
  Kp Stance/1 -> Switch3/1, Switch2/1, Switch1/1, Switch/1
  Demux/1 -> Switch/2
  Switch/1 -> Mux/1
  Mux/1 -> Kp/1
  Stance/Flight [1/0] x4/1 -> Demux/1
  Switch3/1 -> Mux/4
  Switch2/1 -> Mux/3
  Switch1/1 -> Mux/2
  Demux/2 -> Switch1/2
  Demux/3 -> Switch2/2
  Demux/4 -> Switch3/2

== system hardware_atrias_raibert/Control/Actuator Control/SEA Controller (Torque)/dtau_des ==
  x : Inport
  Gain1 : Gain  Gain=1/sample_time
  difference : simulink/Discrete/Difference  ICPrevInput=0.0  InputProcessing=Inherited  OutMin=[]  OutMax=[]  OutDataType=fixdt(1, 16)  OutScaling=2^-10  DoSatur=off
  two_pole_filter : DiscreteTransferFcn  Numerator=[A_lpf_dtau 0 0]  Denominator=[1 B1_lpf_dtau B2_lpf_dtau]  SampleTime=sample_time
  dx/dt : Outport
  wires:
  two_pole_filter/1 -> dx/dt/1
  x/1 -> Gain1/1
  difference/1 -> two_pole_filter/1
  Gain1/1 -> difference/1

== system hardware_atrias_raibert/Control/Actuator Control/SEA Controller (Torque)/filtered_derivative ==
  x : Inport
  Gain1 : Gain  Gain=1/sample_time
  difference : simulink/Discrete/Difference  ICPrevInput=0.0  InputProcessing=Inherited  OutMin=[]  OutMax=[]  OutDataType=fixdt(1, 16)  OutScaling=2^-10  DoSatur=off
  two_pole_filter : DiscreteTransferFcn  Numerator=[A_lpf_accel 0 0]  Denominator=[1 B1_lpf_accel B2_lpf_accel]  SampleTime=sample_time
  dx/dt : Outport
  wires:
  Gain1/1 -> difference/1
  difference/1 -> two_pole_filter/1
  x/1 -> Gain1/1
  two_pole_filter/1 -> dx/dt/1

== system hardware_atrias_raibert/Control/Behavior Control/Contact Estimation/Contact Time ==
  Enable : EnablePort  StatesWhenEnabling=reset  ShowOutputPort=on
  Constant : Constant
  Discrete-Time Integrator : DiscreteIntegrator  IntegratorMethod=Accumulation: Forward Euler  gainval=sample_time  ExternalReset=rising  SampleTime=sample_time  ICPrevOutput=DiscIntNeverNeededParam  ICPrevScaledInput=DiscIntNeverNeededParam
  ts [s] : Outport  InitialOutput=[0]
  wires:
  Constant/1 -> Discrete-Time Integrator/1
  Enable/1 -> Discrete-Time Integrator/2
  Discrete-Time Integrator/1 -> ts [s]/1

== system hardware_atrias_raibert/Control/Behavior Control/Contact Estimation/Last Contact Time ==
  ts [s] : Inport
  Trigger : TriggerPort  TriggerType=falling  PortDimensions=1
  Ts [s] : Outport  InitialOutput=[0]
  wires:
  ts [s]/1 -> Ts [s]/1

== system hardware_atrias_raibert/Control/Behavior Control/Contact Estimation/Leg Torque Measurements ==
  back [rad rad] : Inport
  front [rad rad] : Inport  Port=2
  Demux : Demux  Outputs=2
  Demux1 : Demux  Outputs=2
  Spring Stiffness1 : Gain  Gain=k_sea
  Spring Stiffness2 : Gain  Gain=k_sea
  Sum1 : Sum  Inputs=-+|
  Sum6 : Sum  Inputs=-+|
  Back [Nm] : Outport
  Front [Nm] : Outport  Port=2
  wires:
  Sum6/1 -> Spring Stiffness1/1
  Spring Stiffness1/1 -> Back [Nm]/1
  Sum1/1 -> Spring Stiffness2/1
  Spring Stiffness2/1 -> Front [Nm]/1
  back [rad rad]/1 -> Demux/1
  Demux/2 -> Sum6/2
  Demux/1 -> Sum6/1
  front [rad rad]/1 -> Demux1/1
  Demux1/2 -> Sum1/2
  Demux1/1 -> Sum1/1

== system hardware_atrias_raibert/Control/Behavior Control/Contact Estimation/Vertical Spring Force ==
  theta [rad] : Inport
  phi [rad] : Inport  Port=2
  Force [N] : Inport  Port=3
  Gain : Gain  Gain=-1
  Product : Product
  Sum : Sum  Inputs=++|
  Trigonometric Function : Trigonometry  Operator=cos
  Vertical Force [N] : Outport
  wires:
  Force [N]/1 -> Product/1
  phi [rad]/1 -> Sum/2
  theta [rad]/1 -> Sum/1
  Trigonometric Function/1 -> Product/2
  Product/1 -> Gain/1
  Sum/1 -> Trigonometric Function/1
  Gain/1 -> Vertical Force [N]/1

== system hardware_atrias_raibert/Control/Behavior Control/Lateral PID Control/Lateral Hip PID ==
  position_error : Inport
  velocity_error : Inport  Port=2
  Discrete-Time Integrator : DiscreteIntegrator  IntegratorMethod=Integration: Trapezoidal  SampleTime=sample_time  LimitOutput=on  UpperSaturationLimit=i_limit_lateral  LowerSaturationLimit=-i_limit_lateral  ICPrevOutput=DiscIntNeverNeededParam  ICPrevScaledInput=DiscIntNeverNeededParam
  Sum : Sum  Inputs=+++
  kd_lateral : Gain  Description=xPCTag(1)=kd_lateral;  Gain=kd_lateral
  ki_lateral : Gain  Description=xPCTag(1)=ki_lateral;  Gain=ki_lateral
  kp_lateral : Gain  Description=xPCTag(1)=kp_lateral;  Gain=kp_lateral
  out : Outport
  wires:
  velocity_error/1 -> kd_lateral/1
  Discrete-Time Integrator/1 -> Sum/3
  ki_lateral/1 -> Discrete-Time Integrator/1
  kp_lateral/1 -> Sum/2
  position_error/1 -> ki_lateral/1, kp_lateral/1
  Sum/1 -> out/1
  kd_lateral/1 -> Sum/1

== system hardware_atrias_raibert/Control/Behavior Control/Lateral PID Control/spherical_correction_angle ==
  q_cmu : Inport
  Selector : Selector  InputPortWidth=13  Indices=[11]
  Sum1 : Sum  Inputs=|+-
  Terminator2 : Terminator
  boom_mount_angle : Constant  Value=boom_mount_angle
  lateral_correction : Gain  Gain=180/pi
  lateral_correction [rad] : Outport
  wires:
  Sum1/1 -> lateral_correction/1, lateral_correction [rad]/1
  Selector/1 -> Sum1/1  "qBoomRoll"
  q_cmu/1 -> Selector/1
  boom_mount_angle/1 -> Sum1/2
  lateral_correction/1 -> Terminator2/1

== system hardware_atrias_raibert/Control/Behavior Control/Leg Placement Torque/Leg Angle PD ==
  Desired Angle : Inport
  Desired Velocity : Inport  Port=2
  Leg Angle [rad rad/s] : Inport  Port=3
  Demux1 : Demux  Outputs=2
  Sum7 : Sum  Inputs=|+-
  Sum8 : Sum  Inputs=|+-
  Sum9 : Sum
  kd_leg_angle : Gain  Gain=kd_leg_angle
  kp_leg_angle : Gain  Gain=kp_leg_angle
  Commanded Leg Torque [Nm] : Outport
  wires:
  Leg Angle [rad rad/s]/1 -> Demux1/1
  Demux1/2 -> Sum8/2
  kd_leg_angle/1 -> Sum9/2
  Desired Angle/1 -> Sum7/1
  Sum8/1 -> kd_leg_angle/1
  Desired Velocity/1 -> Sum8/1
  Sum9/1 -> Commanded Leg Torque [Nm]/1
  Demux1/1 -> Sum7/2
  Sum7/1 -> kp_leg_angle/1
  kp_leg_angle/1 -> Sum9/1

== system hardware_atrias_raibert/Control/Behavior Control/Leg Thrust/Thrust Timer ==
  Enable : EnablePort  StatesWhenEnabling=reset  ShowOutputPort=on
  Constant : Constant
  Discrete-Time Integrator : DiscreteIntegrator  IntegratorMethod=Accumulation: Forward Euler  gainval=sample_time  ExternalReset=rising  SampleTime=sample_time  ICPrevOutput=DiscIntNeverNeededParam  ICPrevScaledInput=DiscIntNeverNeededParam
  timer [s] : Outport  InitialOutput=[0]
  wires:
  Discrete-Time Integrator/1 -> timer [s]/1
  Enable/1 -> Discrete-Time Integrator/2
  Constant/1 -> Discrete-Time Integrator/1

== stateflow chart hardware_atrias_raibert/Control/Behavior Control/Raibert  Hopper State Machine ==
  state Loading
    entry: placement = 0;
    entry: posture = 0;
    entry: thrust = 0;
    entry: flight = 0;
    entry: escape = 0;
  state Compression
    entry: placement = 0;
    entry: posture = 1;
    entry: thrust = 0;
    entry: flight = 0;
    entry: escape = 0;
  state Thrust
    entry: placement = 0;
    entry: posture = 1;
    entry: thrust = 1;
    entry: flight = 0;
    entry: escape = 0;
  state Unloading
    entry: placement = 0;
    entry: posture = 0;
    entry: thrust = 1;
    entry: flight = 0;
    entry: escape = 0;
  state Escape
    entry: placement = 0;
    entry: posture = 0;
    entry: thrust = 0;
    entry: flight = 1;
    entry: escape = 1;
  state Flight
    entry: placement = 1;
    entry: posture = 0;
    entry: thrust = 0;
    entry: flight = 1;
    entry: escape = 0;
  (junction 91) -> Loading
  Loading -> (junction 130) [order 2] : [Fy < contact_threshold]
  (junction 93) -> (junction 91)
  (junction 130) -> (junction 128)
  Loading -> Compression [order 1] : [Fy > loaded_threshold]
  (junction 115) -> Compression
  (junction 118) -> (junction 115)
  Compression -> Thrust : [dl >= 0 && dl_prev < 0]
  Thrust -> Unloading [order 1] : [Fy < loaded_threshold]
  Thrust -> (junction 102) [order 2] : [l > l_max]
  (junction 102) -> (junction 100)
  (junction 122) -> (junction 118)
  Unloading -> Escape [order 1] : [Fy < contact_threshold || l > l_max]
  Unloading -> (junction 122) [order 2] : [Fy > loaded_threshold]
  Escape -> Flight : after(t_flight,sec)
  (junction 100) -> Escape
  (default) -> Flight
  Flight -> (junction 93) : [Fy > contact_threshold]
  (junction 128) -> Flight
  data: flight output; escape output; thrust output; posture output; l input; dl input; dl_prev input; Fy input; t_flight parameter; placement output; l_max parameter; contact_threshold parameter; loaded_threshold parameter

== matlab function hardware_atrias_raibert/Control/Behavior Control/Torque Distribution/Motor Torque Saturation Optimization ==
  data: x1s input; t1 output; x2s input; lambda1 parameter; lambda2 parameter; LEG_MTR_MAX_TORQUE parameter; t2 output
% Optimal leg motor torque distribution
function [t1, t2] = distribute_torque(x1s, x2s, lambda1, lambda2, LEG_MTR_MAX_TORQUE)

s = LEG_MTR_MAX_TORQUE;

% possible solutions
x1 = [                                                      x1s;
                                                            0;
                                                            s;
                                                            0;
                                                           -s;
  (lambda2*s + lambda1*x1s - lambda2*x2s)/(lambda1 + lambda2);
  (lambda1*x1s - lambda2*s + lambda2*x2s)/(lambda1 + lambda2);
  (lambda2*s + lambda1*x1s + lambda2*x2s)/(lambda1 + lambda2);
 -(lambda2*s - lambda1*x1s + lambda2*x2s)/(lambda1 + lambda2)];
 
x2 = [                                                      x2s;
                                                            s;
                                                            0;
                                                           -s;
                                                            0;
  (lambda1*s - lambda1*x1s + lambda2*x2s)/(lambda1 + lambda2);
  (lambda1*s + lambda1*x1s + lambda2*x2s)/(lambda1 + lambda2);
  (lambda1*x1s - lambda1*s + lambda2*x2s)/(lambda1 + lambda2);
 -(lambda1*s + lambda1*x1s - lambda2*x2s)/(lambda1 + lambda2)];

% test constraints
c1 = s - x1 - x2 >= 0;
c2 = s + x1 + x2 >= 0;
c3 = s - x1 + x2 >= 0;
c4 = s + x1 - x2 >= 0;
constraints = c1 & c2 & c3 & c4;

% objective function to maximize
f = -lambda1*(x1-x1s).^2-lambda2*(x2-x2s).^2;
satisfied = find(constraints);
[~,I] = max(f(satisfied));

t1 = x1(satisfied(I));
t2 = x2(satisfied(I));

== matlab function hardware_atrias_raibert/Control/Behavior Control/dx_from_yaw_and_roll ==
  data: qRoll input; dx output; dqYaw input; dqPitch input; l_boom parameter; boom_mount_to_center_diagonal parameter; boom_mount_to_com parameter
function dx = fcn(qRoll, dqYaw, dqPitch, l_boom, boom_mount_to_center_diagonal, boom_mount_to_com)
dx = (l_boom+boom_mount_to_center_diagonal)*(dqYaw*cos(qRoll)) - dqPitch*boom_mount_to_com;
